simulink model "Exp5b_Up_Down_Control_Method2"  (R2020a)
settings: Solver=FixedStepAuto  StartTime=0.0  StopTime=10.0  RelTol=1e-3  EnableMultiTasking=on
libraries: arduinolib x3
settings Model: SILPILModeSetting=veronly  ExtModeTrigDuration=2  Creator=jprak  LastModifiedBy=jprak
settings OptimizationCC: EnhancedBackFolding=on  PassReuseOutputArgsAs=Individual arguments  ZeroExternalMemoryAtStartup=off  ZeroInternalMemoryAtStartup=off  MaxStackSize=64  OptimizeBlockOrder=speed  DifferentSizesBufferReuse=on  OptimizationCustomize=off  EfficientTunableParamExpr=on
settings DebuggingCC: ParameterTunabilityLossMsg=error
settings HardwareCC: ProdBitPerInt=16  ProdBitPerPointer=16  ProdBitPerSizeT=16  ProdBitPerPtrDiffT=16  ProdLargestAtomicFloat=None  ProdWordSize=8  ProdHWDeviceType=Atmel->AVR
settings SFSimCC: MATLABDynamicMemAlloc=off
settings RTWCC: SystemTargetFile=ert.tlc  HardwareBoard=Arduino Uno  TLCOptions=-aInlineSetEventsForThisBaseRateFcn=TLC_FALSE -aSuppressMultiTaskScheduler=TLC_FALSE -aRateBasedStepFcn=1  TemplateMakefile=ert_default_tmf  Toolchain=Arduino AVR  BuildConfiguration=Faster Runs
settings CodeAppCC: ForceParamTrailComments=on  IgnoreCustomStorageClasses=off  OperatorAnnotations=on  SimulinkDataObjDesc=on  SFDataObjDesc=on  InsertBlockDesc=on
settings ERTTargetCC: SupportContinuousTime=on  SupportVariableSizeSignals=on  ExtModeStaticAllocSize=250

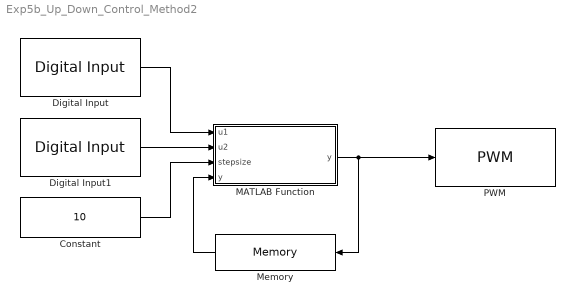
== system Exp5b_Up_Down_Control_Method2 ==
  Constant : Constant  Value=10
  Digital Input : arduinolib/Digital Input  pinNumber=8  Direction=input  SampleTime=0.1  blockPlatform=arduino
  Digital Input1 : arduinolib/Digital Input  pinNumber=7  Direction=input  SampleTime=0.1  blockPlatform=arduino
  MATLAB Function : MATLAB Function  TreatAsAtomicUnit=on
  Memory : Memory
  PWM : arduinolib/PWM  pinNumber=5  frequencyType=Default  desiredFrequency=490.2  achievableFrequency=490.2
  wires:
  Digital Input1/1 -> MATLAB Function/2(u2)
  Digital Input/1 -> MATLAB Function/1(u1)
  Constant/1 -> MATLAB Function/3(stepsize)
  MATLAB Function/1(y) -> PWM/1, Memory/1
  Memory/1 -> MATLAB Function/4("y ")

== matlab function Exp5b_Up_Down_Control_Method2/MATLAB Function ==
  data: u1 input; y output; u2 input; stepsize input; y input
function y = fcn(u1,u2,stepsize,y)
if(u1==1)
    y = min(y+stepize,255);
elseif(u2==1)
    y = max(y-stepsize,0);
else
    y=y;
end
